simulink model "vtol50kg_airframe_ECEF"  (R2024b)
settings: Solver=VariableStepAuto  StartTime=0.0  StopTime=10.0  RelTol=1e-3
undefined symbols (not defined in the file or in its folder): Earth, F, Light, MIL, WGS84, WMM2020
libraries: aerolibasang x5, aerolibwind2 x3, aerolib6dof2 x1, aerolibatmos2 x1, aerolibgravity2 x1
settings Model: Creator=CETCA  LastModifiedBy=CETCA

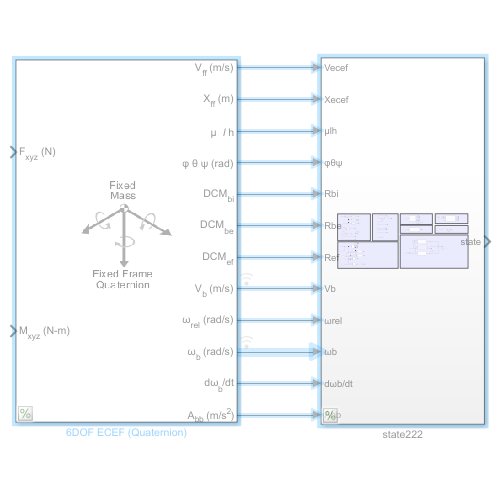
[thumbnail: Simulink's stored preview of the top-level diagram]
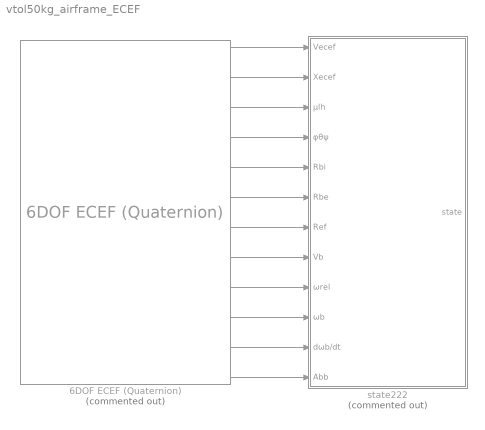
== system vtol50kg_airframe_ECEF ==
  6DOF ECEF (Quaternion) : aerolib6dof2/6DOF ECEF (Quaternion)  Commented=on  units=Metric (MKS)  mtype=Fixed  xg_0=[0 0 0]  Vm_0=plant.init.vx_vy_vz  eul_0=plant.init.phi_theta_psi  pm_0=plant.init.p_q_r  mass_0=1  mass_e=0.5  mass_f=2.0  inertia=eye(3)  inertia_e=eye(3)  inertia_f=2*eye(3)  vre_flag=on  abi_flag=off  ptype=Earth (WGS84)  R=6378137  F=1/298.257223563  w_E=7292115e-11  angle_in=Internal  LPM0=0  quat_statename=''  pm_statename=''  Vm_statename=''  posfixedframe_statename=''  posinertial_statename=''  LPM_statename=''  mass_statename=''
  state222 : Subsystem  Commented=on
  wires:
  6DOF ECEF (Quaternion)/6 -> state222/6(Rbe)
  6DOF ECEF (Quaternion)/8 -> state222/8(Vb)
  6DOF ECEF (Quaternion)/3 -> state222/3(μlh)
  6DOF ECEF (Quaternion)/7 -> state222/7(Ref)
  6DOF ECEF (Quaternion)/9 -> state222/9(ωrel)
  6DOF ECEF (Quaternion)/12 -> state222/12(Abb)
  6DOF ECEF (Quaternion)/1 -> state222/1(Vecef)
  6DOF ECEF (Quaternion)/11 -> state222/11(dωb/dt)
  6DOF ECEF (Quaternion)/5 -> state222/5(Rbi)
  6DOF ECEF (Quaternion)/4 -> state222/4(φθψ)
  6DOF ECEF (Quaternion)/2 -> state222/2(Xecef)
  6DOF ECEF (Quaternion)/10 -> state222/10(ωb)

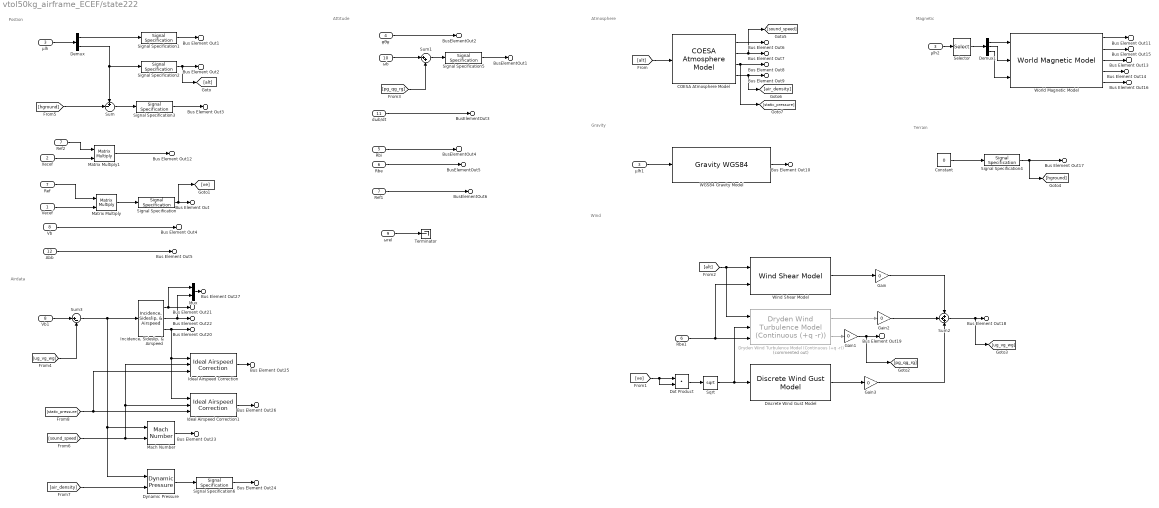
== system vtol50kg_airframe_ECEF/state222 ==
  note: Airdata
  note: Wind
  note: Terrain
  note: Magnetic
  note: Gravity
  note: Atmosphere
  note: Attitude
  note: Postion
  Vecef : Inport
  Xecef : Inport  Port=2
  μlh : Inport  Port=3
  φθψ : Inport  Port=4
  Rbi : Inport  Port=5
  Rbe : Inport  Port=6
  Ref : Inport  Port=7
  Vb : Inport  Port=8
  ωrel : Inport  Port=9
  ωb : Inport  Port=10
  dωb/dt : Inport  Port=11
  Abb : Inport  Port=12
  COESA Atmosphere Model : aerolibatmos2/COESA Atmosphere Model  units=Metric (MKS)  spec=1976 COESA-extended U.S. Standard Atmosphere  model=Profile  profile_var=High temperature  profile_percent=1%  profile_alt=5 km (16404 ft)  envelope_var=High temperature  envelope_percent=1%  action=Warning
  Constant : Constant  Value=0
  Demux : Demux  Outputs=[2 1]
  Demux1 : Demux  Outputs=3
  Discrete Wind Gust Model : aerolibwind2/Discrete Wind Gust Model  units=Metric (MKS)  Gx=on  Gy=on  Gz=on  t_0=5  d_m=[120 120 80]  v_m=[3.5 3.5 3.0]
  Dot Product : DotProduct  OutDataTypeStr=Inherit: Inherit via internal rule
  Dryden Wind Turbulence Model (Continuous (+q -r)) : aerolibwind2/Dryden Wind Turbulence Model  (Continuous (+q -r))  Commented=on  units=Metric (MKS)  spec=MIL-F-8785C  model=Continuous Dryden (+q -r)  W20=15  Wdeg=0  TurbProb=10^-2 - Light  L_high=533.4  Wingspan=10  ts=0.1  Seed=[23341 23342 23343 23344]  T_on=on
  Dynamic Pressure : aerolibasang/Dynamic Pressure
  Gain{,1..3} (4 alike) : Gain  Gain=0
  Ideal Airspeed Correction : aerolibasang/Ideal Airspeed Correction  units=Metric (MKS)  vel_in=TAS  vel_out_tas=CAS  vel_out_eas=TAS  vel_out_cas=TAS  method=Table Lookup  SubOnly=off  action=None
  Ideal Airspeed Correction1 : aerolibasang/Ideal Airspeed Correction  units=Metric (MKS)  vel_in=TAS  vel_out_tas=EAS  vel_out_eas=TAS  vel_out_cas=TAS  method=Table Lookup  SubOnly=off  action=None
  "Incidence, Sideslip, & Airspeed" : aerolibasang/Incidence, Sideslip, & Airspeed
  Mach Number : aerolibasang/Mach Number
  Matrix Multiply : Product  Multiplication=Matrix(*)
  Matrix Multiply1 : Product  Multiplication=Matrix(*)
  Mux : Mux  Inputs=2
  Rbe1 : InportShadow  Port=6
  Ref1 : InportShadow  Port=7
  Ref2 : InportShadow  Port=7
  Selector : Selector  InputPortWidth=3  IndexOptions=Index vector (dialog)  Indices=[3 1 2]  OutputSizes=1
  Signal Specification : SignalSpecification  Unit=m/s
  Signal Specification1 : SignalSpecification  Unit=deg
  Signal Specification2 : SignalSpecification  Unit=m
  Signal Specification3 : SignalSpecification  Unit=m
  Signal Specification4 : SignalSpecification  Unit=m
  Signal Specification5 : SignalSpecification  Unit=rad/s
  Signal Specification6 : SignalSpecification  Unit=Pa
  Sqrt : Sqrt
  Sum : Sum  Inputs=+-|
  Sum1 : Sum  Inputs=|++
  Sum2 : Sum  Inputs=+++
  Sum3 : Sum  Inputs=|+-
  Terminator : Terminator
  Vb1 : InportShadow  Port=8
  "WGS84 Gravity Model  " : GravityWGS84
  Wind Shear Model : aerolibwind2/Wind Shear Model  units=Metric (MKS)  phase=Category C - Terminal Flight Phase  W_20=15  Wdeg=0
  World Magnetic Model : aerolibgravity2/World Magnetic Model  model=WMM2020 (2020-2025)  customFile='WMM2020.COF'  units=Metric (MKS)  time_in=off  month=January  day=1  year=2020  action=Error  h_out=on  dec_out=on  inc_out=on  ti_out=on
  μlh1 : InportShadow  Port=3
  μlh2 : InportShadow  Port=3
  Bus Element Out1 : Outport  PortName=state  Element=aircraft.position.lat_lon
  Bus Element Out2 : Outport  PortName=state  Element=aircraft.position.alt
  Bus Element Out3 : Outport  PortName=state  Element=aircraft.position.agl
  Bus Element Out12 : Outport  PortName=state  Element=aircraft.position.pn_pe_pd
  Bus Element Out : Outport  PortName=state  Element=aircraft.position.vn_ve_vd
  Bus Element Out4 : Outport  PortName=state  Element=aircraft.position.ub_vb_wb
  Bus Element Out5 : Outport  PortName=state  Element=aircraft.position.ax_ay_az
  BusElementOut2 : Outport  PortName=state  Element=aircraft.attitude.phi_theta_psi
  BusElementOut1 : Outport  PortName=state  Element=aircraft.attitude.p_q_r
  BusElementOut3 : Outport  PortName=state  Element=aircraft.attitude.pdot_qdot_rdot
  BusElementOut4 : Outport  PortName=state  Element=aircraft.attitude.Rbi
  BusElementOut5 : Outport  PortName=state  Element=aircraft.attitude.Rbe
  BusElementOut6 : Outport  PortName=state  Element=aircraft.attitude.Ref
  Bus Element Out20 : Outport  PortName=state  Element=aircraft.airdata.airspeed
  Bus Element Out21 : Outport  PortName=state  Element=aircraft.airdata.alpha
  Bus Element Out22 : Outport  PortName=state  Element=aircraft.airdata.beta
  Bus Element Out23 : Outport  PortName=state  Element=aircraft.airdata.mach
  Bus Element Out24 : Outport  PortName=state  Element=aircraft.airdata.qbar
  Bus Element Out25 : Outport  PortName=state  Element=aircraft.airdata.airspeed_cali
  Bus Element Out26 : Outport  PortName=state  Element=aircraft.airdata.airspeed_equ
  Bus Element Out27 : Outport  PortName=state  Element=aircraft.airdata.alpha_beta
  Bus Element Out6 : Outport  PortName=state  Element=environ.atmosphere.temperature
  Bus Element Out7 : Outport  PortName=state  Element=environ.atmosphere.soundspeed
  Bus Element Out8 : Outport  PortName=state  Element=environ.atmosphere.pressure
  Bus Element Out9 : Outport  PortName=state  Element=environ.atmosphere.density
  Bus Element Out10 : Outport  PortName=state  Element=environ.gravity.xyz
  Bus Element Out11 : Outport  PortName=state  Element=environ.magnetic.xyz
  Bus Element Out13 : Outport  PortName=state  Element=environ.magnetic.declination
  Bus Element Out14 : Outport  PortName=state  Element=environ.magnetic.inclination
  Bus Element Out15 : Outport  PortName=state  Element=environ.magnetic.hor_intensity
  Bus Element Out16 : Outport  PortName=state  Element=environ.magnetic.total_intensity
  Bus Element Out17 : Outport  PortName=state  Element=environ.terrain.hground
  Bus Element Out18 : Outport  PortName=state  Element=environ.wind.ug_vg_wg
  Bus Element Out19 : Outport  PortName=state  Element=environ.wind.pg_qg_rg
  wires:
  Ref/1 -> Matrix Multiply/1
  Vecef/1 -> Matrix Multiply/2
  Matrix Multiply/1 -> Signal Specification/1
  Signal Specification/1 -> [ve], Bus Element Out/1
  μlh/1 -> Demux/1
  Demux/1 -> Signal Specification1/1
  Signal Specification1/1 -> Bus Element Out1/1
  Demux/2 -> Signal Specification2/1, Sum/1
  Signal Specification2/1 -> [alt], Bus Element Out2/1
  Sum/1 -> Signal Specification3/1
  Signal Specification3/1 -> Bus Element Out3/1
  [hground] -> Sum/2
  Vb/1 -> Bus Element Out4/1
  Abb/1 -> Bus Element Out5/1
  φθψ/1 -> BusElementOut2/1
  Rbi/1 -> BusElementOut4/1
  Rbe/1 -> BusElementOut5/1
  Ref1/1 -> BusElementOut6/1
  ωb/1 -> Sum1/1
  Sum1/1 -> Signal Specification5/1
  [pg_qg_rg] -> Sum1/2
  dωb/dt/1 -> BusElementOut3/1
  ωrel/1 -> Terminator/1
  Xecef/1 -> Matrix Multiply1/2
  Ref2/1 -> Matrix Multiply1/1
  Matrix Multiply1/1 -> Bus Element Out12/1
  [alt] -> COESA Atmosphere Model/1
  COESA Atmosphere Model/1 -> Bus Element Out6/1
  COESA Atmosphere Model/2 -> [sound_speed], Bus Element Out7/1
  COESA Atmosphere Model/3 -> [static_pressure], Bus Element Out8/1
  COESA Atmosphere Model/4 -> [air_density], Bus Element Out9/1
  μlh1/1 -> "WGS84 Gravity Model  "/1
  "WGS84 Gravity Model  "/1 -> Bus Element Out10/1
  μlh2/1 -> Selector/1
  Selector/1 -> Demux1/1
  Demux1/1 -> World Magnetic Model/1
  Demux1/2 -> World Magnetic Model/2
  Demux1/3 -> World Magnetic Model/3
  World Magnetic Model/1 -> Bus Element Out11/1
  World Magnetic Model/3 -> Bus Element Out13/1
  World Magnetic Model/4 -> Bus Element Out14/1
  World Magnetic Model/2 -> Bus Element Out15/1
  World Magnetic Model/5 -> Bus Element Out16/1
  Constant/1 -> Signal Specification4/1
  Signal Specification4/1 -> [hground], Bus Element Out17/1
  Dryden Wind Turbulence Model (Continuous (+q -r))/1 -> Gain2/1
  Discrete Wind Gust Model/1 -> Gain3/1
  Dryden Wind Turbulence Model (Continuous (+q -r))/2 -> Gain1/1
  Rbe1/1 -> Wind Shear Model/2, Dryden Wind Turbulence Model (Continuous (+q -r))/3
  [alt] -> Wind Shear Model/1, Dryden Wind Turbulence Model (Continuous (+q -r))/1
  [ve] -> Dot Product/2, Dot Product/1
  Dot Product/1 -> Sqrt/1
  Sqrt/1 -> Dryden Wind Turbulence Model (Continuous (+q -r))/2, Discrete Wind Gust Model/1
  Sum2/1 -> [ug_vg_wg], Bus Element Out18/1
  Wind Shear Model/1 -> Gain/1
  Gain1/1 -> [pg_qg_rg], Bus Element Out19/1
  Vb1/1 -> Sum3/1
  [ug_vg_wg] -> Sum3/2
  Sum3/1 -> "Incidence, Sideslip, & Airspeed"/1, Dynamic Pressure/1, Mach Number/1
  "Incidence, Sideslip, & Airspeed"/3 -> Ideal Airspeed Correction/1, Ideal Airspeed Correction1/1, Bus Element Out20/1
  "Incidence, Sideslip, & Airspeed"/2 -> Mux/2, Bus Element Out22/1
  "Incidence, Sideslip, & Airspeed"/1 -> Mux/1, Bus Element Out21/1
  [sound_speed] -> Ideal Airspeed Correction1/2, Ideal Airspeed Correction/2, Mach Number/2
  Mach Number/1 -> Bus Element Out23/1
  Dynamic Pressure/1 -> Signal Specification6/1
  [air_density] -> Dynamic Pressure/2
  [static_pressure] -> Ideal Airspeed Correction/3, Ideal Airspeed Correction1/3
  Ideal Airspeed Correction/1 -> Bus Element Out25/1
  Ideal Airspeed Correction1/1 -> Bus Element Out26/1
  Mux/1 -> Bus Element Out27/1
  Gain/1 -> Sum2/1
  Gain2/1 -> Sum2/2
  Gain3/1 -> Sum2/3
  Signal Specification5/1 -> BusElementOut1/1
  Signal Specification6/1 -> Bus Element Out24/1
